simulink model "BlindSpotComposition"  (R2024b)
settings: Solver=FixedStepDiscrete  StartTime=0.0  StopTime=inf  FixedStep=0.1  RelTol=1e-3
values from neighbouring files (symbols this model uses):
  TurnSignalStatusType : value not decoded    [BlindSpotDataTypes.sldd]
settings Model: DataDictionary=BlindSpotDataTypes.sldd  Creator=Emir  LastModifiedBy=Emir
settings OptimizationCC: DefaultParameterBehavior=Inlined  EnhancedBackFolding=on  PassReuseOutputArgsAs=Individual arguments  ZeroExternalMemoryAtStartup=off  ZeroInternalMemoryAtStartup=off  OptimizeBlockOrder=speed  DifferentSizesBufferReuse=on  OptimizationCustomize=off  EfficientTunableParamExpr=on
settings DebuggingCC: ParameterTunabilityLossMsg=error
settings SFSimCC: MATLABDynamicMemAlloc=off
settings RTWCC: Description=AUTOSAR  SystemTargetFile=autosar.tlc  GenCodeOnly=on  TemplateMakefile=ert_default_tmf  DataTypeReplacement=CDataTypesFixedWidth
settings CodeAppCC: ForceParamTrailComments=on  IgnoreCustomStorageClasses=off  OperatorAnnotations=on  SimulinkDataObjDesc=on  SFDataObjDesc=on  InsertBlockDesc=on
settings STFCustomTargetCC: TargetLangStandard=C99 (ISO)  MultiwordLength=256  ParMdlRefBuildCompliant=on  CompOptLevelCompliant=on  IncludeMdlTerminateFcn=off  CombineOutputUpdateFcns=on  SuppressErrorStatus=on  ERTCustomFileBanners=on  SupportNonFinite=off  SupportComplex=off  SupportContinuousTime=off  SupportNonInlinedSFcns=off  RemoveResetFunc=on  MATLABClassNameForMDSCustomization=Simulink.SoftwareTarget.ERTCustomization  AutosarCompliant=on  UseToolchainInfoCompliant=on  LookupTableObjectStructAxisOrder=2,1,3,4,...  LUTObjectStructOrderEvenSpacing=Size,Table,Breakpoints  SystemTargetFile=autosar.tlc
settings ERTTargetCC: TargetLangStandard=C99 (ISO)  ConcurrentExecutionCompliant=off  IncludeMdlTerminateFcn=off  SuppressErrorStatus=on  SupportNonFinite=off  SupportComplex=off  ModelStepFunctionPrototypeControlCompliant=off  CPPClassGenCompliant=off  AutosarCompliant=on  LookupTableObjectStructAxisOrder=2,1,3,4,...  LUTObjectStructOrderEvenSpacing=Size,Table,Breakpoints  ERTCustomFileTemplate=example_file_process.tlc  BooleanTrueId=TRUE  BooleanFalseId=FALSE

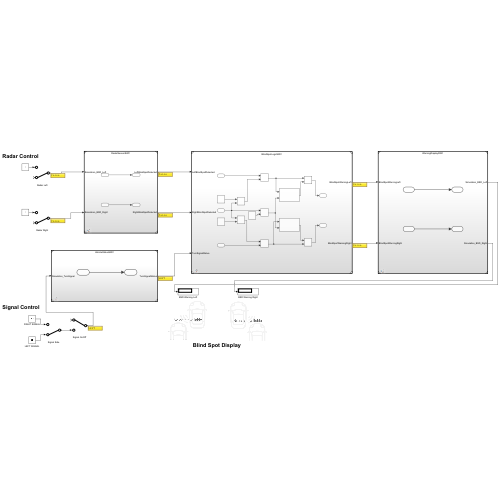
[thumbnail: Simulink's stored preview of the top-level diagram]
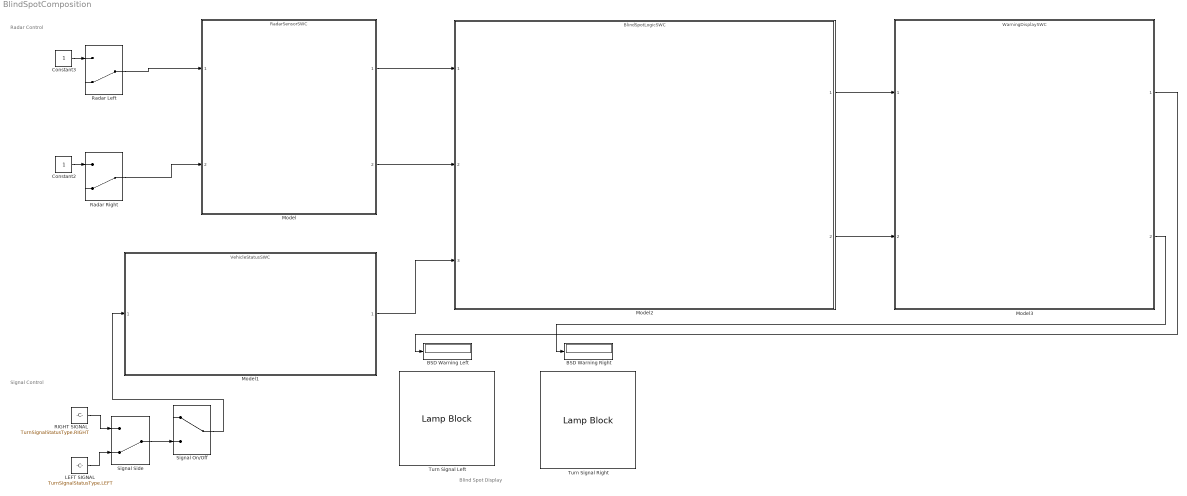
== system BlindSpotComposition ==
  note: Signal Control
  note: Radar Control
  note: Blind Spot Display
  BSD Warning Left : Display
  BSD Warning Right : Display
  Constant2 : Constant  OutDataTypeStr=BlindSpotDetectedType
  Constant3 : Constant  OutDataTypeStr=BlindSpotDetectedType
  LEFT SIGNAL : Constant  Value=TurnSignalStatusType.LEFT  OutDataTypeStr=Enum: TurnSignalStatusType
  Model : ModelReference  ModelNameDialog=RadarSensorSWC.slx  SimulationMode=Normal  ModelReferenceVersion=1.9
  Model1 : ModelReference  ModelNameDialog=VehicleStatusSWC.slx  SimulationMode=Normal  ModelReferenceVersion=1.10
  Model2 : ModelReference  ModelNameDialog=BlindSpotLogicSWC.slx  SimulationMode=Normal  ModelReferenceVersion=1.18
  Model3 : ModelReference  ModelNameDialog=WarningDisplaySWC.slx  SimulationMode=Normal  ModelReferenceVersion=1.8
  RIGHT SIGNAL : Constant  Value=TurnSignalStatusType.RIGHT  OutDataTypeStr=Enum: TurnSignalStatusType
  Radar Left : ManualSwitch  CurrentSetting=0
  Radar Right : ManualSwitch  CurrentSetting=0
  Signal On/Off : ManualSwitch
  Signal Side : ManualSwitch  CurrentSetting=0
  Turn Signal Left : LampBlock  LabelPosition=Hide  Icon=Custom  CustomIcon=data:image/svg+xml;base64,PD94bWwgdmVyc2lvbj0iMS4wIiBzdGFuZGFsb25lPSJubyI/Pgo8IURPQ1RZUEUgc3ZnIFBVQkxJQyAiLS8vVzNDLy9EVEQgU1ZHIDIwMDEwOTA0Ly9FTiIKICJodHRwOi8vd3d3LnczLm9yZy9UUi8yMDAxL1JFQy1TVkctMjAwMTA5MDQvRFREL3N2ZzEwLmR0ZCI+CjxzdmcgdmVyc2lvbj0iMS4wIiB4bWxucz0iaHR0cDovL3d3dy53My5vcmcvMjAwMC9zdmciCiB3aWR0aD0iNTEyLjAwMDAwMHB0IiBoZWlnaHQ9IjUxMi4wMDAwMDBwdCIgdmlld0JveD0iMCAwIDUxMi4wMDAwMDAgNTEyLjAwMDAwMCIKIHByZXNlcnZlQXNwZWN0 ...(+5956 chars)
  Turn Signal Right : LampBlock  LabelPosition=Hide  Icon=Custom  CustomIcon=data:image/svg+xml;base64,PD94bWwgdmVyc2lvbj0iMS4wIiBzdGFuZGFsb25lPSJubyI/Pgo8IURPQ1RZUEUgc3ZnIFBVQkxJQyAiLS8vVzNDLy9EVEQgU1ZHIDIwMDEwOTA0Ly9FTiIKICJodHRwOi8vd3d3LnczLm9yZy9UUi8yMDAxL1JFQy1TVkctMjAwMTA5MDQvRFREL3N2ZzEwLmR0ZCI+CjxzdmcgdmVyc2lvbj0iMS4wIiB4bWxucz0iaHR0cDovL3d3dy53My5vcmcvMjAwMC9zdmciCiB3aWR0aD0iNTEyLjAwMDAwMHB0IiBoZWlnaHQ9IjUxMi4wMDAwMDBwdCIgdmlld0JveD0iMCAwIDUxMi4wMDAwMDAgNTEyLjAwMDAwMCIKIHByZXNlcnZlQXNwZWN0 ...(+6060 chars)
  wires:
  Model/1 -> Model2/1
  Model/2 -> Model2/2
  Model1/1 -> Model2/3
  Model2/2 -> Model3/2
  Model2/1 -> Model3/1
  Model3/1 -> BSD Warning Left/1
  Model3/2 -> BSD Warning Right/1
  RIGHT SIGNAL/1 -> Signal Side/1
  LEFT SIGNAL/1 -> Signal Side/2
  Signal Side/1 -> Signal On/Off/2
  Signal On/Off/1 -> Model1/1
  Constant2/1 -> Radar Right/1
  Constant3/1 -> Radar Left/1
  Radar Right/1 -> Model/2
  Radar Left/1 -> Model/1
